simulink model "Model_4a_CH4_constant_clean"  (R2019a)
settings: Solver=FixedStepAuto  StartTime=0.0  StopTime=8760  FixedStep=1  RelTol=1e-3
libraries: simulink x5
settings Model: Creator=senja  LastModifiedBy=senja

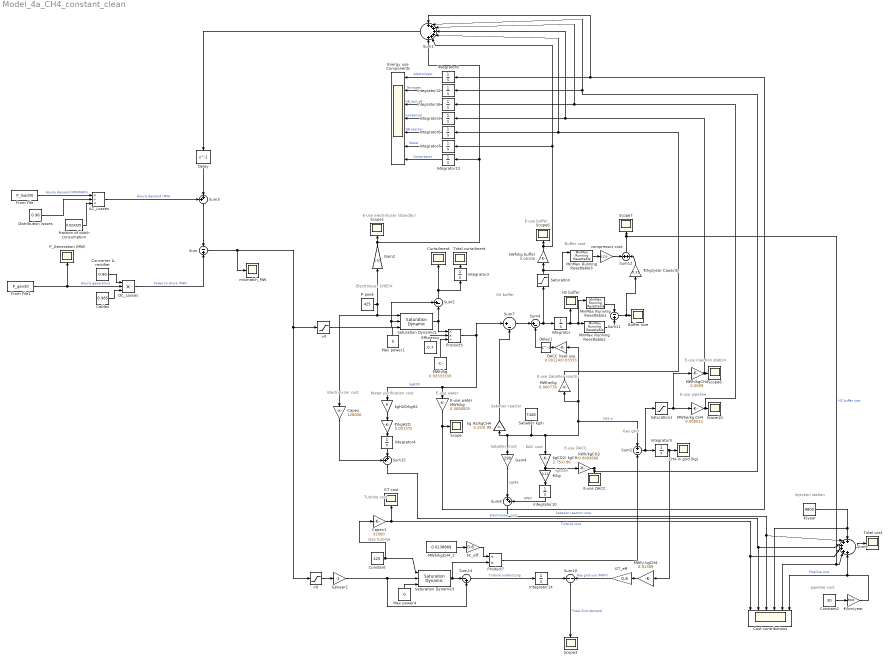
== system Model_4a_CH4_constant_clean ==
  note: DAC cost
  note: Water purification cost
  note: E-use pipeline
  note: pipeline cost
  note: E-use injection station
  note: E-use buffer
  note: Buffer cost
  note: E-use Sabatier reactor
  note: E-use DACC
  note: Sabatier_Cost
  note: Injection station
  note: Gas grid
  note: Sabatier reactor
  note: E-use electrolyser (standby)
  note: E-use water
  note: Turbine cost
  note: Gas turbine
  note: Electrolyser CHECK
  note: Electrolyzer cost
  note: H2 buffer
  <0 : Saturate  UpperLimit=inf  LowerLimit=0
  >0 : Saturate  UpperLimit=inf  LowerLimit=0
  AC_Losses : Product  Inputs=*/*
  Buffer size : Scope
  CH4 in grid (kg) : Scope
  Cables : Constant  Value=0.985
  Capex : Gain  Gain=126000
  Capex1 : Gain  Gain=32000
  Constant : Constant  Value=425
  Constant2 : Constant  Value=30
  Converter & rectifier : Constant  Value=0.90
  Cost contributions : Scope  NumInputPorts=6
  Curtailment : Scope
  DACC heat use : Gain  Gain=0.00124/0.03333
  DC_Losses : Product  Inputs=3
  Delay : Delay  DelayLength=1  InitialCondition=0
  Delay1 : Delay  DelayLength=1
  Distribution losses : Constant  Value=0.96
  E-use DACC : Scope
  E-use water MWh/kg : Gain  Gain=0.0000005
  Efficiency : Constant  Value=0.7
  Energy use Components : Scope  NumInputPorts=7
  FC_eff. : Gain  Gain=0.6
  From File : FromFile  FileName=P_load30  SampleTime=0
  From File1 : FromFile  FileName=P_gen30  SampleTime=0
  GJ/year1 : Gain  Gain=-1
  GT cost : Scope
  GT_eff : Gain  Gain=0.6
  Gain2 : Gain  Gain=0.02
  Gain4 : Gain  Gain=290
  H2 buffer : Scope
  Integrator{,2..8,10..14} (13 alike) : Integrator
  MWh/ kgCH4 : Gain  Gain=0.01389
  MWh/kg : Constant  Value=0.03333333
  MWh/kgCH4 : Gain  Gain=0.0009
  MWh/kgCH4_2 : Constant  Value=0.0138889
  MWhe/kg : Gain  Gain=0.000778
  MWhe/kg CH4 : Gain  Gain=0.000012
  Max power1 : Constant  Value=0
  Max power4 : Constant  Value=0
  MinMax Running Resettable1 : simulink/Math Operations/MinMax Running Resettable  Function=min  vinit=0.0
  MinMax Running Resettable2 : simulink/Math Operations/MinMax Running Resettable  Function=max  vinit=0.0
  MinMax Running Resettable3 : simulink/Math Operations/MinMax Running Resettable  Function=max  vinit=0.0
  P peek : Constant  Value=425
  P_Generation (MW) : Scope
  Product3 : Product  Inputs=**/
  Product7 : Product  Inputs=/*
  Sabatier kg/h : Constant  Value=7448
  Saturation : Saturate  UpperLimit=inf  LowerLimit=0
  Saturation Dynamic1 : simulink/Discontinuities/Saturation Dynamic  OutMin=[]  OutMax=[]  OutDataTypeStr=Inherit: Same as second input  OutDataType=fixdt(1, 16)  OutScaling=2^-10  DoSatur=off
  Saturation Dynamic3 : simulink/Discontinuities/Saturation Dynamic  OutMin=[]  OutMax=[]  OutDataTypeStr=Inherit: Same as second input  OutDataType=fixdt(1, 16)  OutScaling=2^-10  DoSatur=off
  Saturation1 : Saturate  UpperLimit=inf  LowerLimit=0
  Scope{,1,3,6..8,10} (7 alike) : Scope
  Sum : Sum  Inputs=-|+
  Sum1 : Sum  Inputs=+++++++
  Sum10 : Sum  Inputs=-|-
  Sum11 : Sum  Inputs=-|+
  Sum12 : Sum  Inputs=+|+
  Sum14 : Sum  Inputs=|-+
  Sum15 : Sum  Inputs=++|
  Sum2 : Sum  Inputs=+|-
  Sum3 : Sum  Inputs=++|
  Sum4 : Sum  Inputs=|+-
  Sum5 : Sum  Inputs=+-|
  Sum7 : Sum  Inputs=|+-
  Sum8 : Sum  Inputs=|++
  Sum9 : Sum  Inputs=++++++
  Total cost : Scope
  Total curtailment : Scope
  compressor cost : Gain  Gain=1170
  fraction of dutch consumption : Constant  Value=0.023335
  kWh/kg buffer : Gain  Gain=0.00106
  kWh/kgCO2 : Gain  Gain=0.0003666
  kg H2/kgCH4 : Gain  Gain=0.25/0.96
  kgCO2/ kgCH4 : Gain  Gain=2.75/0.96
  kgH2O/kgH2 : Gain  Gain=9
  mismatch_MW : Scope
  €/kg : Gain  Gain=0.11
  €/kg/year Capacity : Gain  Gain=0.31
  €/kgH2O : Gain  Gain=0.001375
  €/km/year : Gain  Gain=9000
  €/year : Constant  Value=9800
  wires:
  From File/1 -> AC_Losses/1  "Hourly demand (MW/MWh)"
  Efficiency/1 -> Product3/2
  fraction of dutch consumption/1 -> AC_Losses/3
  Distribution losses/1 -> AC_Losses/2
  Cables/1 -> DC_Losses/3
  Converter & rectifier/1 -> DC_Losses/1
  DC_Losses/1 -> Sum/2  "Power to shore (MW)"
  >0/1 -> Sum5/1, Saturation Dynamic1/2
  <0/1 -> GJ/year1/1
  AC_Losses/1 -> Sum3/1  "Hourly demand (MW)"
  From File1/1 -> P_Generation (MW)/1, DC_Losses/2  "Hourly generation"
  Max power1/1 -> Saturation Dynamic1/3
  Saturation Dynamic1/1 -> Sum5/2, Product3/1
  Capex/1 -> Sum15/1
  Sum15/1 -> Sum9/3, Cost contributions/2  "Electrolyzer  cost"
  €/kgH2O/1 -> Integrator4/1
  P peek/1 -> Saturation Dynamic1/1, Capex/1, Gain2/1
  GJ/year1/1 -> Saturation Dynamic3/2, Sum14/2
  Product3/1 -> Sum7/1, kgH2O/kgH2/1, E-use water MWh/kg/1  "kgH2/h"
  Sum/1 -> <0/1, >0/1, mismatch_MW/1
  Sum9/1 -> Total cost/1
  Constant/1 -> Saturation Dynamic3/1, Capex1/1
  Max power4/1 -> Saturation Dynamic3/3
  Saturation Dynamic3/1 -> Product7/2, Sum14/1
  MWh/kgCH4_2/1 -> FC_eff./1
  Integrator3/1 -> Total curtailment/1
  kgH2O/kgH2/1 -> €/kgH2O/1
  Integrator4/1 -> Sum15/2
  MWh/kg/1 -> Product3/3
  Capex1/1 -> Cost contributions/1, Sum9/4, GT cost/1  "Turbine cost"
  FC_eff./1 -> Product7/1
  Sum5/1 -> Integrator3/1, Curtailment/1
  Sum14/1 -> Integrator14/1  "Turbine undersizing"
  E-use water MWh/kg/1 -> Integrator8/1, Sum1/1, Scope/1
  Gain2/1 -> Scope1/1, Sum1/7, Integrator13/1
  Sum3/1 -> Sum/1
  Sum1/1 -> Delay/1
  Delay/1 -> Sum3/2
  Integrator2/1 -> Energy use Components/4  "condenser"
  Integrator6/1 -> Energy use Components/5  "HB reactor"
  Integrator7/1 -> Energy use Components/6  "Water"
  Integrator8/1 -> Energy use Components/1  "electrolyser"
  Product7/1 -> Sum2/2
  Integrator/1 -> MinMax Running Resettable1/1, MinMax Running Resettable2/1, H2 buffer/1
  Sum10/1 -> Scope3/1  "Total Grid demand"
  MWh/ kgCH4/1 -> GT_eff/1
  GT_eff/1 -> Sum10/2  "Gas grid use (MWh)"
  Integrator5/1 -> CH4 in grid (kg)/1, MWh/ kgCH4/1
  Gain4/1 -> Sum8/1  "CAPEX"
  kgCO2/ kgCH4/1 -> kWh/kgCO2/1, €/kg/1  "kgCO2/h"
  €/kg/1 -> Integrator10/1
  Sum8/1 -> Sum9/2, Cost contributions/3  "Sabatier reactorr cost"
  Integrator10/1 -> Sum8/2  "OPEX"
  MWhe/kg/1 -> Sum1/5, Integrator6/1
  Integrator12/1 -> Energy use Components/2  "Nitrogen"
  Integrator11/1 -> Energy use Components/3  "HB_boil off"
  kWh/kgCO2/1 -> E-use DACC/1, Sum1/2, Integrator12/1
  MinMax Running Resettable1/1 -> Sum11/1
  MinMax Running Resettable2/1 -> Sum11/2
  Sum11/1 -> Buffer size/1, €/kg/year Capacity/1
  €/kg/year Capacity/1 -> Sum12/2
  kWh/kg buffer/1 -> Sum1/6, Integrator7/1, Scope6/1
  Saturation/1 -> kWh/kg buffer/1, MinMax Running Resettable3/1
  MinMax Running Resettable3/1 -> compressor cost/1
  compressor cost/1 -> Sum12/1
  Sum12/1 -> Scope7/1, Sum9/5, Cost contributions/5  "H2 buffer cost"
  Integrator13/1 -> Energy use Components/7  "Compressor"
  Sum2/1 -> Saturation1/1, Integrator5/1
  €/year/1 -> Cost contributions/4, Sum9/1
  Saturation1/1 -> MWh/kgCH4/1, MWhe/kg CH4/1
  MWh/kgCH4/1 -> Sum1/4, Integrator2/1, Scope8/1
  Constant2/1 -> €/km/year/1
  €/km/year/1 -> Cost contributions/6, Sum9/6  "Pipeline cost"
  MWhe/kg CH4/1 -> Sum1/3, Integrator11/1, Scope10/1
  Integrator14/1 -> Sum10/1
  kg H2/kgCH4/1 -> Sum7/2
  DACC heat use/1 -> Delay1/1
  Delay1/1 -> Sum4/2
  Sabatier kg/h/1 -> DACC heat use/1, MWhe/kg/1, Sum2/1, kgCO2/ kgCH4/1, kg H2/kgCH4/1, Gain4/1  "CH4 in"
  Sum7/1 -> Sum4/1
  Sum4/1 -> Integrator/1, Saturation/1
